simulink model "assign3_test1"  (R2020b)
settings: Solver=VariableStepAuto  StartTime=0.0  StopTime=20  RelTol=1e-3
values from neighbouring files (symbols this model uses):
  A = [4,1,-2;1,0,2;1,-1,3]    [test.m]    (also in test2.m = [1 0 0 0;2 -3 0 0;1 0 -2 0;4 -1 -2 -4]; test3.m = [-1 0 0 0;2 -3 0 0;0 0 2 0;4 -1 2 -4])
  B = [3,1;2,7;5,3]    [test.m]    (also in test2.m = [0;0;1;2]; test3.m = [0 0 1 2]')
  C = [1,2,0;0,1,1]    [test.m]    (also in test2.m = [3 0 1 0]; test3.m = [3 0 1 0])
  D = [0,0;0,0]    [test.m]    (also in test3.m = [0])
  G = tf(num,den)    [test.m]    (also in test3.m = inv(To1)*Go)
  K = [0 0 K1(1) K1(2)]*Tc1    [test3.m]
settings Model: Creator=10911  LastModifiedBy=10911

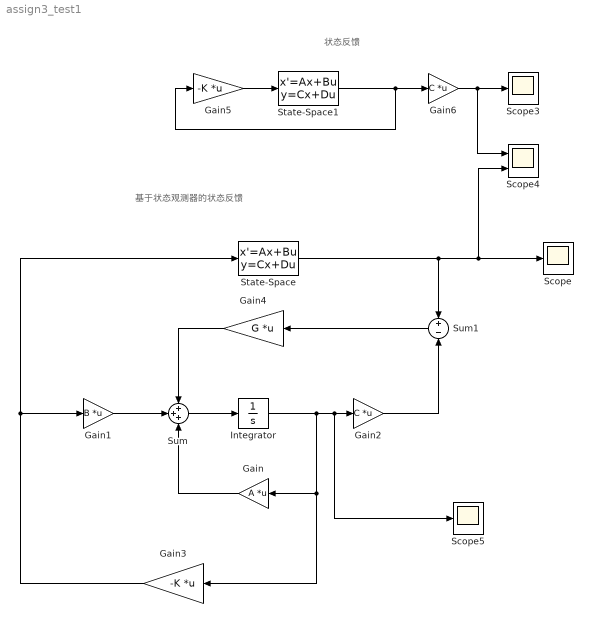
== system assign3_test1 ==
  note: 状态反馈
  note: 基于状态观测器的状态反馈
  Gain : Gain  Gain=A  Multiplication=Matrix(K*u)
  Gain1 : Gain  Gain=B  Multiplication=Matrix(K*u)
  Gain2 : Gain  Gain=C  Multiplication=Matrix(K*u)
  Gain3 : Gain  Gain=-K  Multiplication=Matrix(K*u)
  Gain4 : Gain  Gain=G  Multiplication=Matrix(K*u)
  Gain5 : Gain  Gain=-K  Multiplication=Matrix(K*u)
  Gain6 : Gain  Gain=C  Multiplication=Matrix(K*u)
  Integrator : Integrator  InitialCondition=[0.05 0.1 0.1 0.1]
  Scope : Scope
  Scope3 : Scope
  Scope4 : Scope  NumInputPorts=2
  Scope5 : Scope
  State-Space : StateSpace  A=A  B=B  C=C  D=D  InitialCondition=[0.1 0.2 0.3 0.4]
  State-Space1 : StateSpace  A=A  B=B  C=[1 0 0 0;0 1 0 0;0 0 1 0;0 0 0 1]  D=[0;0;0;0]  InitialCondition=[0.1 0.2 0.3 0.4]
  Sum : Sum  Inputs=+++
  Sum1 : Sum  Inputs=+|-
  wires:
  State-Space/1 -> Scope4/2, Scope/1, Sum1/1
  Sum/1 -> Integrator/1
  Integrator/1 -> Gain3/1, Gain/1, Scope5/1, Gain2/1
  Gain2/1 -> Sum1/2
  Gain/1 -> Sum/3
  Gain1/1 -> Sum/2
  Sum1/1 -> Gain4/1
  Gain3/1 -> State-Space/1, Gain1/1
  Gain4/1 -> Sum/1
  State-Space1/1 -> Gain6/1, Gain5/1
  Gain5/1 -> State-Space1/1
  Gain6/1 -> Scope4/1, Scope3/1
